simulink model "test3"  (R2018b)
settings: Solver=FixedStepAuto  StartTime=0.0  StopTime=20  FixedStep=0.001  RelTol=1e-3
settings Model: Creator=User  LastModifiedBy=User

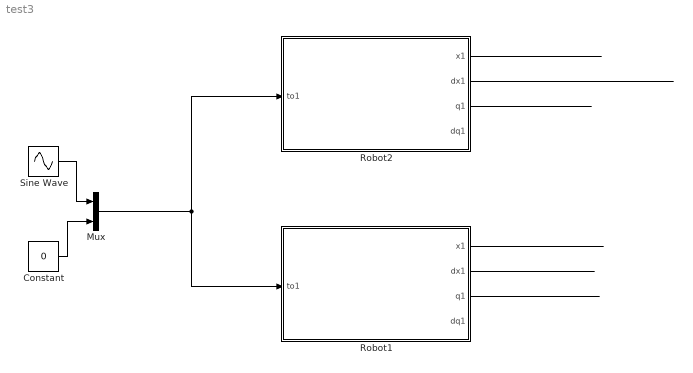
== system test3 ==
  Constant : Constant  Value=0
  Mux : Mux  Inputs=2
  Robot1 : Subsystem
  Robot2 : Subsystem
  Sine Wave : Sin  Amplitude=0.5  Frequency=2*pi  SampleTime=0
  wires:
  Robot2/1(x1) -> ?
  Robot1/1(x1) -> ?
  Sine Wave/1 -> Mux/1
  Constant/1 -> Mux/2
  Mux/1 -> Robot2/1(to1), Robot1/1(to1)
  Robot2/3(q1) -> ?
  Robot1/3(q1) -> ?
  Robot2/2(dx1) -> ?
  Robot1/2(dx1) -> ?

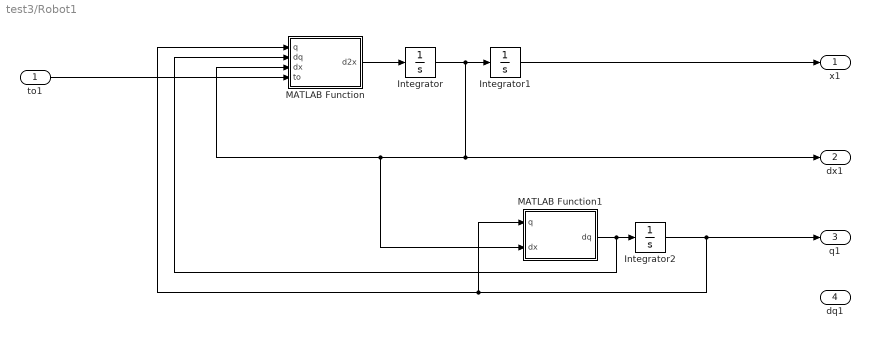
== system test3/Robot1 ==
  to1 : Inport
  Integrator : Integrator  InitialCondition=[0;0]
  Integrator1 : Integrator  InitialCondition=[-3;-2]
  Integrator2 : Integrator  InitialCondition=[pi/6;pi/6]
  MATLAB Function : MATLAB Function  TreatAsAtomicUnit=on
  MATLAB Function1 : MATLAB Function  TreatAsAtomicUnit=on
  x1 : Outport
  dx1 : Outport  Port=2
  q1 : Outport  Port=3
  dq1 : Outport  Port=4
  wires:
  Integrator/1 -> MATLAB Function1/2(dx), MATLAB Function/3(dx), dx1/1, Integrator1/1
  MATLAB Function/1(d2x) -> Integrator/1
  to1/1 -> MATLAB Function/4(to)
  Integrator1/1 -> x1/1
  MATLAB Function1/1(dq) -> MATLAB Function/2(dq), Integrator2/1
  Integrator2/1 -> MATLAB Function/1(q), MATLAB Function1/1(q), q1/1

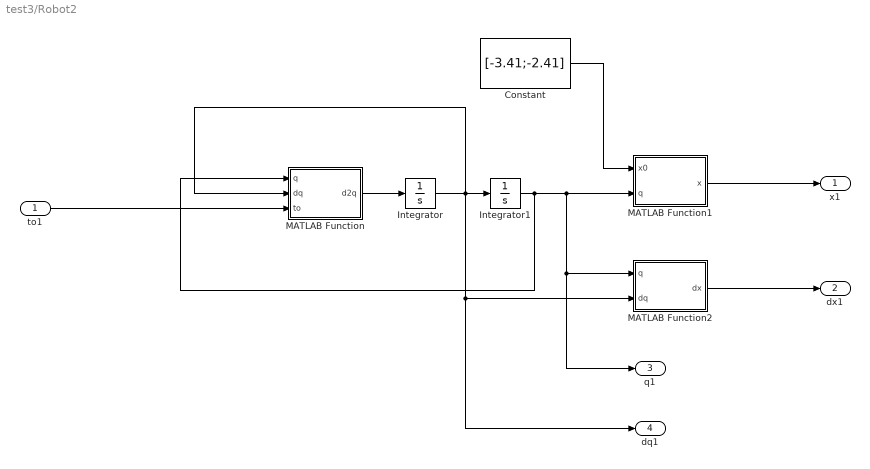
== system test3/Robot2 ==
  to1 : Inport
  Constant : Constant  Value=[-3.41;-2.41]
  Integrator : Integrator  InitialCondition=[0;0]
  Integrator1 : Integrator  InitialCondition=[pi/6;pi/6]
  MATLAB Function : MATLAB Function  TreatAsAtomicUnit=on
  MATLAB Function1 : MATLAB Function  TreatAsAtomicUnit=on
  MATLAB Function2 : MATLAB Function  TreatAsAtomicUnit=on
  x1 : Outport
  dx1 : Outport  Port=2
  q1 : Outport  Port=3
  dq1 : Outport  Port=4
  wires:
  to1/1 -> MATLAB Function/3(to)
  MATLAB Function/1(d2q) -> Integrator/1
  Integrator/1 -> dq1/1, MATLAB Function2/2(dq), MATLAB Function/2(dq), Integrator1/1
  Integrator1/1 -> q1/1, MATLAB Function2/1(q), MATLAB Function1/2(q), MATLAB Function/1(q)
  MATLAB Function1/1(x) -> x1/1
  Constant/1 -> MATLAB Function1/1(x0)
  MATLAB Function2/1(dx) -> dx1/1

== matlab function test3/Robot1/MATLAB Function ==
  data: q input; d2x output; dq input; dx input; to input
function d2x = fcn(q,dq,dx,to)
m1=1;
m2=1;
l1=0.3;
l2=0.3;
t1=1/3*m1*l1^2+m2*l1^2;
t2=1/3*m2*l2^2;
t3=1/2*m2*l1*l2;
t4=0.07;
q1=q(1);
q2=q(2);
Hq=[t1+t2+2*t3*cos(q2) t2+t3*cos(q2);
    t2+t3*cos(q2) t2];
dq1=dq(1);
dq2=dq(2);
Cq=[-dq2*t3*sin(q2) -(dq1+dq2)*t3*sin(q2);
    dq1*t3*sin(q2) 0];
Fq=[t4*dq1;t4*dq2];
J=[-0.3*sin(q1)-0.3*sin(q1+q2) -0.3*sin(q1+q2);
    0.3*cos(q1)+0.3*cos(q1+q2) 0.3*cos(q1+q2)];
dJ=[-0.3*dq1*cos(q1)-0.3*(dq1+dq2)*cos(q1+q2) -0.3*(dq1+dq2)*cos(q1+q2);
    -0.3*dq1*sin(q1)-0.3*(dq1+dq2)*sin(q1+q2) -0.3*(dq1+dq2)*sin(q1+q2)];
Hx=Hq*pinv(J);
Cx=Cq*pinv(J)-Hq*pinv(J)*dJ*pinv(J);
d2x=Hx\(to-Cx*dx-Fq);
end

== matlab function test3/Robot1/MATLAB Function1 ==
  data: q input; dq output; dx input
function dq = fcn(q,dx)
q1=q(1);
q2=q(2);
J=[-0.3*sin(q1)-0.3*sin(q1+q2) -0.3*sin(q1+q2);
    0.3*cos(q1)+0.3*cos(q1+q2) 0.3*cos(q1+q2)];
dq=inv(J)*dx;
end

== matlab function test3/Robot2/MATLAB Function ==
  data: q input; d2q output; dq input; to input
function d2q = fcn(q,dq,to)
m1=1;
m2=1;
l1=0.3;
l2=0.3;
t1=1/3*m1*l1^2+m2*l1^2;
t2=1/3*m2*l2^2;
t3=1/2*m2*l1*l2;
t4=0.07;
q2=q(2);
M=[t1+t2+2*t3*cos(q2) t2+t3*cos(q2);
    t2+t3*cos(q2) t2];
dq1=dq(1);
dq2=dq(2);
Cq=[-dq2*t3*sin(q2) -(dq1+dq2)*t3*sin(q2);
    dq1*t3*sin(q2) 0];
Fq=[t4*dq1;t4*dq2];
d2q=M\(to-Cq*dq-Fq);
end

== matlab function test3/Robot2/MATLAB Function1 ==
  data: x0 input; x output; q input
function x = fcn(x0,q)
q1=q(1);
q2=q(2);
x=x0+[0.3*cos(q1)+0.3*cos(q1+q2);0.3*sin(q1)+0.3*sin(q1+q2)];
end

== matlab function test3/Robot2/MATLAB Function2 ==
  data: q input; dq input; dx output
function dx = fcn(q,dq)
q1=q(1);
q2=q(2);
J=[-0.3*sin(q1)-0.3*sin(q1+q2) -0.3*sin(q1+q2);
    0.3*cos(q1)+0.3*cos(q1+q2) 0.3*cos(q1+q2)];
dx=J*dq;
end
